simulink model "motor_config"  (R2025a)
settings: Solver=FixedStepAuto  StartTime=0.0  StopTime=inf  FixedStep=Ts  RelTol=1e-3
undefined symbols (not defined in the file): MAX_FORCE, MAX_SPEED, OPERATION_MODE
settings Model: Creator=AKZW  LastModifiedBy=AKZW
settings OptimizationCC: LocalBlockOutputs=off
settings SFSimCC: UsePrecompiledLibraries=Avoid
settings RTWCC: SystemTargetFile=TwinCatGrt.tlc  GenCodeOnly=on  GenerateMakefile=off  TemplateMakefile=tcgrt_msbuild.tmf  TargetLang=C++  Description=TwinCAT GRT Target
settings STFCustomTargetCC: SystemTargetFile=TwinCatGrt.tlc  TargetLangStandard=C++11 (ISO)  MultiwordLength=2048.0  DynamicStringBufferSize=256.0  ConcurrentExecutionCompliant=on  CombineOutputUpdateFcns=on  CodeInterfacePackaging=Reusable function  CPPClassGenCompliant=on  GRTInterface=off  GenerateAllocFcn=on  TcPlcFb_MonitorExecutionTime=off  TcCom_DataStoreReadOnly=off  TcCom_ModuleCaller=CyclicTask  TcProject_PublishConfiguration=Release  TcCom_ContStateReadOnly=on  TcCom_InputCreateSymbols=on  TcCom_BlockDiagramVariableAccess=AssignToParent  TcProject_VendorIcon=$<TE140x:Icon>  TcCom_VariableSymbolMapping=Identical  TcCom_InitExceptionHandling=CallerExceptions  TcProject_PreferIntOverLong=off  TcCom_GroupName=TE140x|Simulink Modules  TcProject_BuildWithWdk=inherit default  TcCom_BlockIoCreateSymbols=on  TcProject_GenerateVsSolution=No  TcProject_PublishTcUMx86=off  TcProject_EnableNewPlatforms=off  TcProject_CreateScopedEnums=Auto  TcPlcFb_ExtModeRtAllowExecutionCommands=off  TcProject_PublishTcOSx64E=off  TcProject_ClassFactoryName=$<Project:Name>  TcPlcFb_OemLicenses=$<Project:OemLicenses>  TcCom_ExtModeRtAllowForParameterChange=off  TcCom_ParametersDataAccess=Internal DataArea  TcCom_ExecuteModelCode=on  TcProject_InstallPlcLibrary=off  TcProject_LowestCompatibleTcBuild=$<TwinCAT:Version:BUILD>  TcCom_ModuleIcon=$<TE140x:Icon>  TcProject_LibraryCategories=$<VendorName>  TcCom_VariableSymbolMappingCustom=$<ModelName>_U=Input|$<ModelName>_Y=Output|$<ModelName>_P=ModelParameters|$<ModelName>_B=BlockIO|$<ModelName>_DW=DWork|$<ModelName>_X=ContStates  TcProject_VendorName=TE140x Module Vendor  TcPlcFb_InitExceptionHandling=CallerExceptions  TcCom_GroupIcon=$<TE140x:Icon>  TcCom_ExtModeRtAllowExecutionCommands=off  TcCom_TcComWrapperFbProperties=off  TcProject_Generate=on  TcProject_GenerateStructDutsWithDefaultValues=Auto  TcProject_Copyright=Copyright $<VendorName> $<LocalDateTime:%Y>  TcProject_Versioning=Versioned  TcProject_PreferToolArchitectureX64=on  TcCom_GroupDisplayName=$<GroupName>  TcProject_PublishTcOSARMv7A=off  TcProject_ProductName=$<ModuleGenerator:ProductId> $<ModuleGenerator:Version:MAJOR.MINOR>  TcCom_ParametersCreateSymbols=on  TcCom_DWorkReadOnly=on  TcCom_TcComWrapperFbPropertyMonitoring=NoMonitoring  TcProject_GeneratePlcLibrary=off  TcCom_AllowDataAreaForSharedData=off  TcCom_OnlineChangeRestoreDataAreas=off  TcProject_PublishParallel=on  TcCom_DataStoreDataAccess=None  TcCom_StrictAccessLock=on  TcCom_GlobalParamDefaultSharing=Define  TcCom_ExtModeRtWaitForStart=off  TcCom_MonitorExecutionTime=off  TcProject_PublishTcOSARMv8A=off  TcProject_UseDataExchangeModules=off  TcCom_ContStateCreateSymbols=on  TcProject_PublishTcOSARMv7M=off  TcProject_Description=TwinCAT executable file, generated by TwinCAT $<ModuleGenerator:ProductId>  TcCom_InputInitValues=off  TcCom_StepSizeAdaptation=RequireMatchingTaskCycleTime  TcProject_UseCodeInfoExporter=on  TcProject_UseCodeDescriptor=on  TcPlcFb_UpdateExceptionHandling=CallerExceptions  TcCom_MaxInternalDataAreaParts=5U  TcProject_UseTmxExtension=Auto  TcProject_MaxVisibleArrayElements=200U  TcCom_DataStoreCreateSymbols=on  TcCom_OutputReadOnly=on  TcProject_PublishPlatformtoolset=Auto  TcProject_DrvFileVersion=$<VersionFromFile>  TcCom_AccessLockState=Auto  TcProject_StaticStlStringCapacity=Auto  TcProject_UseStaticStlString=off  TcProject_SignWithTwinCatCertificate=inherit default  TcProject_IgnorePseudoArrayDimensions=off  TcProject_UseNativeBlockDiagramExport=off  TcProject_CreateUniqueEnumItemNames=off  TcCom_ContStateDataAccess=Internal DataArea  TcCom_BlockIoReadOnly=on  TcCom_OutputDataAccess=Output Source DataArea  TcCom_OnlineChange=off  TcProject_PublishTcOSx64=off  TcProject_PublishTcRTx64=on  TcCom_InputDataAccess=Input Destination DataArea  TcCom_ResolveMaskedSubsystems=on  TcProject_PlcVarPrefixes=PVOID=p | BOOL=b | BOOL32=b | DATE=d | TIME_OF_DATE=td | TIME=t | LTIME=t | GUID=n  TcCom_DWorkDataAccess=Internal DataArea  TcCom_BlockDiagramDebugInfoExport=on  TcProject_ForceRebuildForPublish=off  TcProject_VersionSrc=$<LatestTMFile>  TcProject_LibCatPath=$<Project:Dir>\$<Project:Name>.libcat.xml  TcProject_UseIntrinsics=on  TcProject_SignTwinCatCertName=TcTestCert  TcProject_IncrementVersion=Revision  TcCom_OriginalIoBlockNames=off  TcCom_ExecutionSequence=UpdateBeforeOutputMapping  TcProject_PublishTcRTx86=on  TcCom_ExtendSignalResolution=off  TcCom_OemLicenses=$<Project:OemLicenses>  TcProject_TmxInstall=on  TcProject_UseDescriptorCodeType=on  TcProject_CoderCppNamespace=coder  TcProject_CLanguageStandard=Default  TcProject_CppLanguageStandard=Default  TcCom_DWorkCreateSymbols=on  TcCom_InputReadOnly=off  TcProject_UseLLVMCodeInfo=on  TcCom_ParametersReadOnly=off  TcCom_ExecutionInfoOutput=off  TcCom_UpdateExceptionHandling=CallerExceptions  TcProject_Publish=on  TcPlcFb_ExtModeRtAllowForParameterChange=off  TcCom_TcComWrapperFb=off  TcProject_DataExchangeModulesVersion=$<ModuleGenerator:DataExchange:Version>  TcPlcFb_Generate=off  TcCom_Generate=on  TcCom_OutputCreateSymbols=on  TcProject_DeployRestart=off  TcProject_BuildSystem=Auto  TcProject_Verbosity=Normal  TcCom_BlockIoDataAccess=Internal DataArea  TcCom_ExecutionInfoParam=on  TcCom_BlockDiagramExport=on  TcCom_CallerVerification=Default  TcCom_Legacy_ModuleBuildInfoParam=on  TcProject_PublishTcUMx64=off  TcProject_DrvProductVersion=$<DrvFileVersion>  TcPlcFb_ExtModeRtWaitForStart=off  TcCom_ParametersInitValues=on
settings GRTTargetCC: ExtModeMexFile=TcExtModeClient  TargetLangStandard=C++11 (ISO)  ParMdlRefBuildCompliant=off  CompOptLevelCompliant=off  MatFileLogging=off  CodeInterfacePackaging=Reusable function  GenerateAllocFcn=on  UseToolchainInfoCompliant=off

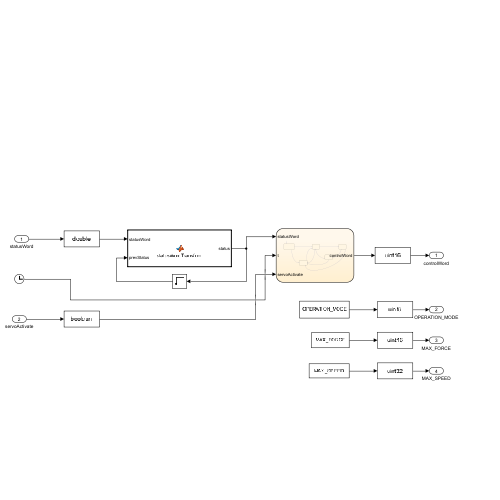
[thumbnail: Simulink's stored preview of the top-level diagram]
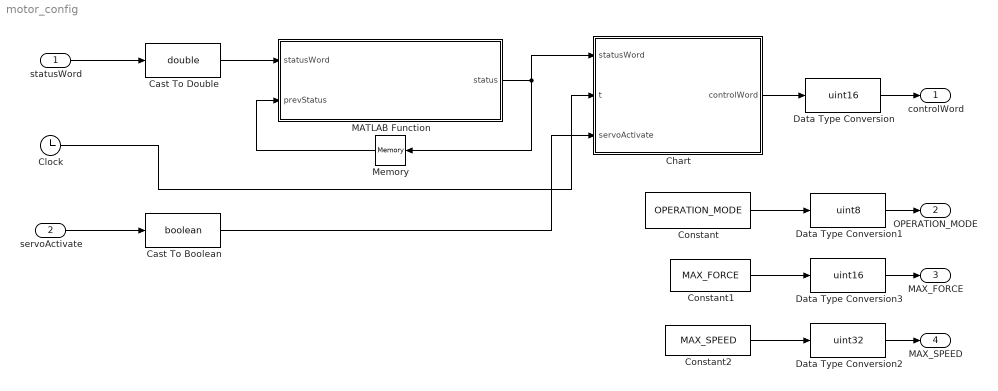
== system motor_config ==
  statusWord : Inport  OutDataTypeStr=uint16
  servoActivate : Inport  Port=2
  Cast To Boolean : DataTypeConversion  OutDataTypeStr=boolean  SaturateOnIntegerOverflow=off  RndMeth=Floor
  Cast To Double : DataTypeConversion  OutDataTypeStr=double  SaturateOnIntegerOverflow=off  RndMeth=Floor
  Chart : Stateflow chart  TreatAsAtomicUnit=on
  Clock : Clock
  Constant : Constant  Value=OPERATION_MODE
  Constant1 : Constant  Value=MAX_FORCE
  Constant2 : Constant  Value=MAX_SPEED
  Data Type Conversion : DataTypeConversion  OutDataTypeStr=uint16  SaturateOnIntegerOverflow=off  RndMeth=Floor
  Data Type Conversion1 : DataTypeConversion  OutDataTypeStr=uint8  SaturateOnIntegerOverflow=off  RndMeth=Floor
  Data Type Conversion2 : DataTypeConversion  OutDataTypeStr=uint32  SaturateOnIntegerOverflow=off  RndMeth=Floor
  Data Type Conversion3 : DataTypeConversion  OutDataTypeStr=uint16  SaturateOnIntegerOverflow=off  RndMeth=Floor
  MATLAB Function : MATLAB Function  TreatAsAtomicUnit=on
  Memory : Memory
  controlWord : Outport  VectorParamsAs1DForOutWhenUnconnected=off
  OPERATION_MODE : Outport  Port=2  VectorParamsAs1DForOutWhenUnconnected=off
  MAX_FORCE : Outport  Port=3  VectorParamsAs1DForOutWhenUnconnected=off
  MAX_SPEED : Outport  Port=4  VectorParamsAs1DForOutWhenUnconnected=off
  wires:
  Data Type Conversion2/1 -> MAX_SPEED/1
  Chart/1(controlWord) -> Data Type Conversion/1
  statusWord/1 -> Cast To Double/1
  servoActivate/1 -> Cast To Boolean/1
  Cast To Double/1 -> MATLAB Function/1(statusWord)
  Data Type Conversion1/1 -> OPERATION_MODE/1
  Data Type Conversion/1 -> controlWord/1
  Data Type Conversion3/1 -> MAX_FORCE/1
  Cast To Boolean/1 -> Chart/3(servoActivate)
  Clock/1 -> Chart/2(t)
  Constant1/1 -> Data Type Conversion3/1
  MATLAB Function/1(status) -> Chart/1(statusWord), Memory/1
  Constant2/1 -> Data Type Conversion2/1
  Constant/1 -> Data Type Conversion1/1
  Memory/1 -> MATLAB Function/2(prevStatus)

== matlab function motor_config/MATLAB Function ==
  data: statusWord input; status output; prevStatus input
function status = statusWordTransform(statusWord, prevStatus)

    % Define status codes as constants
    STATUS_NOT_READY_TO_SWITCH_ON = 0; % 0x0000
    STATUS_SWITCH_ON_DISABLED = 64; % 0x0040
    STATUS_READY_TO_SWITCH_ON = 33; % 0x0021
    STATUS_SWITCHED_ON = 35; % 0x0023
    STATUS_OPERATION_ENABLED = 39; % 0x0027
    STATUS_FAULT = 8; % 0x0008
    STATUS_FAULT_REACTION_ACTIVE = 16; % 0x0010
    STATUS_QUICK_STOP_ACTIVE = 7; % 0x0007

    % Save status codes to a MAT file for Simulink usage
    STATUS_CODES = struct(...
      'NOT_READY_TO_SWITCH_ON', STATUS_NOT_READY_TO_SWITCH_ON, ...
      'SWITCH_ON_DISABLED', STATUS_SWITCH_ON_DISABLED, ...
      'READY_TO_SWITCH_ON', STATUS_READY_TO_SWITCH_ON, ...
      'SWITCHED_ON', STATUS_SWITCHED_ON, ...
      'OPERATION_ENABLED', STATUS_OPERATION_ENABLED, ...
      'FAULT', STATUS_FAULT, ...
      'FAULT_REACTION_ACTIVE', STATUS_FAULT_REACTION_ACTIVE, ...
      'QUICK_STOP_ACTIVE', STATUS_QUICK_STOP_ACTIVE ...
    );


    stateList = [ ...
        STATUS_CODES.SWITCH_ON_DISABLED, ...
        STATUS_CODES.READY_TO_SWITCH_ON, ...
        STATUS_CODES.SWITCHED_ON, ...
        STATUS_CODES.OPERATION_ENABLED, ...
        STATUS_CODES.FAULT ...
    ];

    for i = 1:numel(stateList)
        if bitand(statusWord, stateList(i)) == stateList(i) && prevStatus ~= stateList(i)
            status = stateList(i);
            return;
        end
    end

    % どれにも該当しない場合
    status = STATUS_CODES.SWITCHED_ON;
end

== stateflow chart motor_config/Chart ==
  state NotReadyToSwitchOn
    controlWord=0;
  state SwitchOnDisabled
    controlWord=6;
  state SwitchedON
    controlWord=7;
  state OperationEnable
    controlWord=15;
  state Error
    during:
    controlWord = 128
  (default) -> NotReadyToSwitchOn
  NotReadyToSwitchOn -> SwitchOnDisabled [order 1] : [statusWord == 64 && t >= 2]
  SwitchOnDisabled -> SwitchedON [order 1] : [statusWord==33 && servoActivate == 1]
  Error -> SwitchOnDisabled : [after(3,sec)]
  SwitchedON -> Error [order 2] : [statusWord==8]
  SwitchOnDisabled -> Error [order 2] : [statusWord==8]
  OperationEnable -> SwitchOnDisabled [order 1] : [servoActivate==0]
  SwitchedON -> OperationEnable [order 1] : [statusWord == 35]
  NotReadyToSwitchOn -> Error [order 2] : [statusWord==8]
  OperationEnable -> Error [order 2] : [statusWord==8]
  data: statusWord input; t input; controlWord output; servoActivate input
